simulink model "delta_PIDF"  (R2020b)
settings: Solver=VariableStepAuto  StartTime=0.0  StopTime=10  RelTol=1e-3
model workspace: external: MATLAB File robot_delta_DataFile.m (data not in the file)
values from neighbouring files (symbols this model uses):
  smiData = struct    [smi.m]
undefined symbols (not defined in the file or in its folder): _STEP_SLDPRT, lower_leg_1, lower_leg_2, X, Y, Z
libraries: sm_lib x85, fl_lib x26, nesl_utility x16, ee_lib x9, pid_lib x6, fuzblock x3, Multibody_Multiphysics_Lib x3
(part 4 of 4)

== system delta_PIDF/Motor_3/Joint Servo/Fuzzy PID ==
  e : Inport
  Demux : Demux  Outputs=3
  Fuzzy Logic Controller : fuzblock/Fuzzy Logic  Controller  FIS='Fuzzy_PID'  OutputSampleNumber=101  DataType=double  FuzzifiedInputs=off  RuleFiringStrengths=off  RuleOutputs=off  AggregatedOutputs=off  SimulateUsing=Interpreted execution  OutOfRangeInputValueMessage=warning  NoRuleFiredMessage=warning  EmptyOutputFuzzySetMessage=warning
  Mux : Mux  Inputs=2
  Mux2 : Mux  Inputs=3
  N : Constant  Value=300
  PID Controller1 : pid_lib/PID Controller  Controller=PID  Form=Parallel  TimeDomain=Continuous-time  UseExternalTs=off  SampleTime=-1  IntegratorMethod=Forward Euler  FilterMethod=Forward Euler  ControllerParametersSource=external  P=0.6*4.6737  I=1.2*4.6737/3.26  D=0.6*4.6737*3.26/8  UseFilter=on  N=100  TunerSelectOption=Transfer Function Based (PID Tuner App)  InitialConditionSource=internal  InitialConditionForIntegrator=0  InitialConditionForFilter=0  DifferentiatorICPrevScaledInput=0  ExternalReset=none  TrackingMode=off  Kt=1  LimitOutput=off  SatLimitsSource=internal  UpperSaturationLimit=inf  LowerSaturationLimit=-inf  LinearizeAsGain=on  AntiWindupMode=none  Kb=1  POutMin=[]  POutMax=[]  IOutMin=[]  IOutMax=[]  DOutMin=[]  DOutMax=[]  NOutMin=[]  NOutMax=[]  SumOutMin=[]  SumOutMax=[]  SaturationOutMin=[]  SaturationOutMax=[]  PParamMin=[]  PParamMax=[]  IParamMin=[]  IParamMax=[]  DParamMin=[]  DParamMax=[]  NParamMin=[]  NParamMax=[]  KbParamMin=[]  KbParamMax=[]  KtParamMin=[]  KtParamMax=[]  KbOutMin=[]  KbOutMax=[]  KtOutMin=[]  KtOutMax=[]  IntegratorOutMin=[]  IntegratorOutMax=[]  FilterOutMin=[]  FilterOutMax=[]  SumI1OutMin=[]  SumI1OutMax=[]  SumI2OutMin=[]  SumI2OutMax=[]  SumI3OutMin=[]  SumI3OutMax=[]  SumI4OutMin=[]  SumI4OutMax=[]  SumDOutMin=[]  SumDOutMax=[]  DifferentiatorOutMin=[]  DifferentiatorOutMax=[]  FilterDiffOutCoefMin=[]  FilterDiffOutCoefMax=[]  ReciprocalOutMin=[]  ReciprocalOutMax=[]  SumDenOutMin=[]  SumDenOutMax=[]  SumNumOutMin=[]  SumNumOutMax=[]  DivideOutMin=[]  DivideOutMax=[]  UdiffTsProdOutMin=[]  UdiffTsProdOutMax=[]  NTsProdOutMin=[]  NTsProdOutMax=[]  UintegralTsProdOutMin=[]  UintegralTsProdOutMax=[]  UngainTsProdOutMin=[]  UngainTsProdOutMax=[]  IntegratorContinuousStateAttributes=''  IntegratorStateMustResolveToSignalObject=off  IntegratorRTWStateStorageClass=Auto  FilterContinuousStateAttributes=''  FilterStateMustResolveToSignalObject=off  FilterRTWStateStorageClass=Auto  ParallelPVariant=ExternalParameters  IdealPVariant=Disabled  IVariant=ExternalParameters  DVariant=ExternalParameters  IntegratorVariant=Continuous  SatVariant=Disabled  AWVariant=Passthrough  PCopyVariant=Disabled  TRVariant=Disabled  FdbkBlocksVariant=Forward  IdealPFdbkVariant=Disabled  SatFdbkVariant=Disabled  DerivativeFilterVariant=ContFilter  NVariant=ExternalParameters  NCopyVariant=Disabled  FilterICVariant=InternalICsFilter  IntegratorICVariant=InternalICs  ExternalResetVariant=Disabled  TRSumVariant=Passthrough  SumFdbkVariant=Disabled  SumVariant=Sum_PID  TsampFilterVariant=InternalTs  TsampNgainVariant=Passthrough  TsampIntegralVariant=Passthrough  ExternalSaturationOutDataTypeStr=Inherit: Same as second input
  Scope : Scope
  Sum : Sum  Inputs=+-|
  To Workspace : ToWorkspace  VariableName=P3  SampleTime=1
  To Workspace1 : ToWorkspace  VariableName=I3  SampleTime=1
  To Workspace2 : ToWorkspace  VariableName=D3  SampleTime=1
  Unit Delay : UnitDelay  SampleTime=-1  HasFrameUpgradeWarning=on
  u : Outport  VectorParamsAs1DForOutWhenUnconnected=off
  wires:
  PID Controller1/1 -> u/1
  e/1 -> PID Controller1/1, Sum/1, Mux/1, Unit Delay/1
  N/1 -> PID Controller1/5
  Mux/1 -> Fuzzy Logic Controller/1
  Fuzzy Logic Controller/1 -> Demux/1
  Demux/1 -> To Workspace/1, Mux2/1, PID Controller1/2
  Demux/2 -> To Workspace1/1, Mux2/2, PID Controller1/3
  Sum/1 -> Mux/2
  Unit Delay/1 -> Sum/2
  Mux2/1 -> Scope/1
  Demux/3 -> Mux2/3, To Workspace2/1, PID Controller1/4  "alpha"

== matlab function delta_PIDF/MATLAB Function1 ==
  data: t input; out output
function out = rfsignal(t)
L=200;
l=296;
T=5;
ty=1;
d=200;
R=200;
wb=100;
sb=6*wb/sqrt(3);
ub=sqrt(3)*sb/3;
up=50;
sp=up*3/sqrt(3);
wp=sqrt(3)*sp/6;
a=wb-up;
b=sp/2-(sqrt(3)/2)*wb;
c=wp-1/2*wb;

out1=30;out2=30;out3=30;
%z0=-200*sind(out1)-sqrt(296^2-(200*cosd(30)+50)^2)
z0=-d*sind(out1)-sqrt(l^2-(R*cosd(out1)+up)^2)
x=0;y=0;z=z0;

%chay theo duong thang y=-20 x=0 z=z0 trong 1s
if t <= 1
    x=0;y=0;z=z0;
    out=zeros(3,1);
    out(1)=30;
    out(2)=30;
    out(3)=30;
elseif t>1 && t <= (ty+1)
    y=-d/ty*(t-1);
    E1=2*L*(y+a);
    F=2*z*L;
    G1=x^2+y^2+z^2+a^2+L^2+2*y*a-l^2;
    E2=-L*(sqrt(3)*(x+b)+y+c);
    G2=x^2+y^2+z^2+b^2+c^2+L^2+2*(x*b+y*c)-l^2;
    E3=L*(sqrt(3)*(x-b)-y-c);
    G3=x^2+y^2+z^2+b^2+c^2+L^2+2*(-x*b+y*c)-l^2;
    t1=(-F-sqrt(E1^2+F^2-G1^2))/(G1-E1);
    out=zeros(3,1);
    out(1)=2*atand(t1)
    t2=(-F-sqrt(E2^2+F^2-G2^2))/(G2-E2);
    out(2)=2*atand(t2)
    t3=(-F-sqrt(E3^2+F^2-G3^2))/(G3-E3);
    out(3)=2*atand(t3)
else
    y=R*sind(360*t/T-234);
    x=R*cosd(360*t/T-234);
    E1=2*L*(y+a);
    F=2*z*L;
    G1=x^2+y^2+z^2+a^2+L^2+2*y*a-l^2;
    E2=-L*(sqrt(3)*(x+b)+y+c);
    G2=x^2+y^2+z^2+b^2+c^2+L^2+2*(x*b+y*c)-l^2;
    E3=L*(sqrt(3)*(x-b)-y-c);
    G3=x^2+y^2+z^2+b^2+c^2+L^2+2*(-x*b+y*c)-l^2;
    t1=(-F-sqrt(E1^2+F^2-G1^2))/(G1-E1);
    out=zeros(3,1);
    out(1)=2*atand(t1)
    t2=(-F-sqrt(E2^2+F^2-G2^2))/(G2-E2);
    out(2)=2*atand(t2)
    t3=(-F-sqrt(E3^2+F^2-G3^2))/(G3-E3);
    out(3)=2*atand(t3)
end
end
